simulink model "stepperMotorADRCSecondOrder"  (R2025a)
settings: Solver=FixedStepDiscrete  StartTime=0.0  StopTime=.4  FixedStep=1/50e6  RelTol=1e-3
undefined symbols (not defined in the file): ADC_Emulated_conversion_factor, alpha_iqd, alpha_ts, b_ts, beta_iqd, beta_ts, biq, Bm, DiscIntNeverNeededParam, gam_iqd, gam_ts, inverseADC_Emulated_Conversion_factor, inverseVoltagetoADCValue, J, k1_iqd, k1_ts, L, PsiM, PWMVoltage, r, RadiansPerCount, RT, Shunt_Amp_Offset, simParams, stepTime, theta_ref, TL, VoltagetoADCValue, vs
libraries: mcbeeMathTransformLib x2
settings Model: Creator=mike  LastModifiedBy=Caleb
settings OptimizationCC: BlockReduction=off  ConditionallyExecuteInputs=off  DefaultParameterBehavior=Inlined
settings HardwareCC: ProdBitPerPointer=32.0  ProdBitPerSizeT=32.0  ProdBitPerPtrDiffT=32.0  ProdLargestAtomicFloat=None  ProdIntDivRoundTo=Undefined  ProdEndianess=Unspecified  ProdWordSize=32.0  ProdHWDeviceType=ASIC/FPGA->ASIC/FPGA  TargetBitPerPointer=64.0  TargetBitPerSizeT=64.0  TargetBitPerPtrDiffT=64.0  TargetLongLongMode=on  TargetIntDivRoundTo=Zero  TargetEndianess=LittleEndian  TargetWordSize=64.0  TargetHWDeviceType=Custom Processor->MATLAB Host Computer  ProdEqTarget=off
settings RTWCC: GPUComputeCapability=3.5

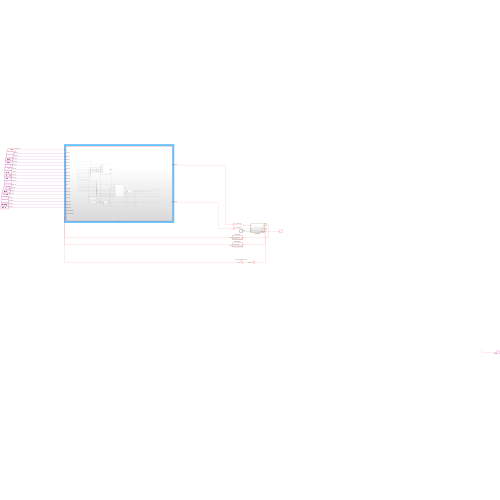
[thumbnail: Simulink's stored preview of the top-level diagram]
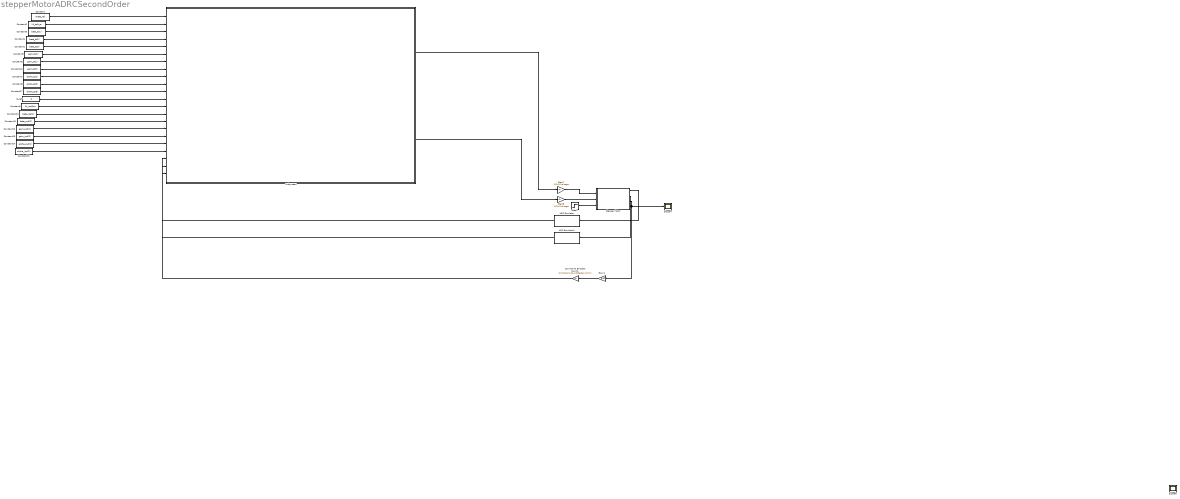
== system stepperMotorADRCSecondOrder ==
  ADC Emulator : Subsystem
  ADC Emulator1 : Subsystem
  Constant : Constant  Value=theta_ref  OutDataTypeStr=fixdt(1,16,8)  SampleTime=-1
  Constant1 : Constant  Value=beta_ts(3)  OutDataTypeStr=fixdt(1,16,8)
  Constant10 : Constant  Value=beta_iqd(1)  OutDataTypeStr=fixdt(1,16,8)
  Constant11 : Constant  Value=beta_iqd(2)  OutDataTypeStr=fixdt(1,16,8)
  Constant12 : Constant  Value=gam_iqd(1)  OutDataTypeStr=fixdt(1,16,8)
  Constant13 : Constant  Value=gam_iqd(2)  OutDataTypeStr=fixdt(1,16,8)
  Constant14 : Constant  Value=alpha_iqd(1)  OutDataTypeStr=fixdt(1,16,8)
  Constant15 : Constant  Value=alpha_iqd(2)  OutDataTypeStr=fixdt(1,16,8)
  Constant16 : Constant  Value=gam_ts(3)  OutDataTypeStr=fixdt(1,16,8)
  Constant17 : Constant  Value=alpha_ts(3)  OutDataTypeStr=fixdt(1,16,8)
  Constant2 : Constant  Value=k1_ts/b_ts  OutDataTypeStr=fixdt(1,16,8)
  Constant3 : Constant  Value=beta_ts(1)  OutDataTypeStr=fixdt(1,16,8)
  Constant4 : Constant  Value=beta_ts(2)  OutDataTypeStr=fixdt(1,16,8)
  Constant5 : Constant  Value=gam_ts(1)  OutDataTypeStr=fixdt(1,16,8)
  Constant6 : Constant  Value=gam_ts(2)  OutDataTypeStr=fixdt(1,16,8)
  Constant7 : Constant  Value=alpha_ts(1)  OutDataTypeStr=fixdt(1,16,8)
  Constant8 : Constant  Value=alpha_ts(2)  OutDataTypeStr=fixdt(1,16,8)
  Constant9 : Constant  Value=k1_iqd/biq  OutDataTypeStr=fixdt(1,16,8)
  Convert To Encoder Counts : Gain  Gain=simParams.CountsPerRev/(2*pi)  OutDataTypeStr=int32
  Gain1 : Gain  Gain=1/RT
  Gain2 : Gain  Gain=1/PWMVoltage  ParamDataTypeStr=fixdt(1,16,8)  OutDataTypeStr=fixdt(1,20,18)
  Gain3 : Gain  Gain=1/PWMVoltage  ParamDataTypeStr=fixdt(1,16,8)  OutDataTypeStr=fixdt(1,20,18)
  Scope4 : Scope
      settings: DataLoggingVariableName=ScopeData4
  Scope6 : Scope
      settings: DataLoggingVariableName=ScopeData6
  Step1 : Step  Time=stepTime  After=TL  SampleTime=0
  Stepper Motor : Subsystem
  Subsystem : Subsystem
  id_ref : Constant  Value=0  OutDataTypeStr=fixdt(1,16,8)
  wires:
  Gain1/1 -> Convert To Encoder Counts/1
  Gain2/1 -> Stepper Motor/1(va)
  Gain3/1 -> Stepper Motor/2(vb)
  Stepper Motor/3(theta_r) -> Scope4/1, Gain1/1
  Stepper Motor/2(ib) -> ADC Emulator1/1(ib)
  Step1/1 -> Stepper Motor/3(TL)
  Stepper Motor/1(ia) -> ADC Emulator/1(ia)
  ? -> Scope6/1
  Constant/1 -> Subsystem/1(r1)
  Constant2/1 -> Subsystem/2(K1_ts/b_ts)
  Constant3/1 -> Subsystem/3(beta_ts(1))
  Constant4/1 -> Subsystem/4(beta_ts(2))
  Constant1/1 -> Subsystem/5(beta_ts(3))
  Constant5/1 -> Subsystem/6(gam_ts(1))
  Constant6/1 -> Subsystem/7(gam_ts(2))
  Constant16/1 -> Subsystem/8(gam_ts(3))
  Constant7/1 -> Subsystem/9(alpha_ts(1))
  Constant8/1 -> Subsystem/10(alpha_ts(2))
  Constant17/1 -> Subsystem/11(alpha_ts(3))
  id_ref/1 -> Subsystem/12(id_ref)
  Constant9/1 -> Subsystem/13(k1_iqd/biq)
  Constant10/1 -> Subsystem/14(beta_iqd(1))
  Constant11/1 -> Subsystem/15(beta_iqd(2))
  Constant12/1 -> Subsystem/16(gam_iqd(1))
  Constant13/1 -> Subsystem/17(gam_iqd(2))
  Constant14/1 -> Subsystem/18(alpha_iqd(1))
  Constant15/1 -> Subsystem/19(alpha_iqd(2))
  ADC Emulator/1(ADC Current Value) -> Subsystem/20(ADC Current Value)
  ADC Emulator1/1(ADC Current Value) -> Subsystem/21(ADC Current Value1)
  Convert To Encoder Counts/1 -> Subsystem/22(In22)
  Subsystem/1(Out1) -> Gain2/1
  Subsystem/2(Out2) -> Gain3/1

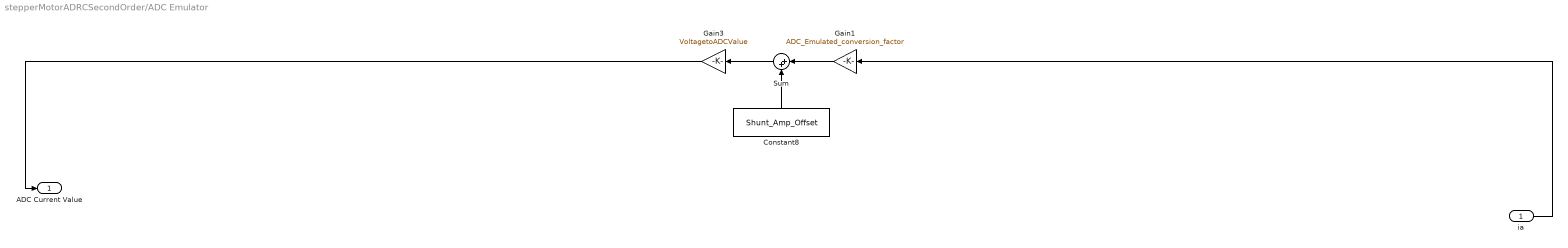
== system stepperMotorADRCSecondOrder/ADC Emulator ==
  ia : Inport
  Constant8 : Constant  Value=Shunt_Amp_Offset  OutDataTypeStr=fixdt(1,16,8)
  Gain1 : Gain  Gain=ADC_Emulated_conversion_factor  ParamDataTypeStr=fixdt(1,16,8)
  Gain3 : Gain  Gain=VoltagetoADCValue  ParamDataTypeStr=int16  OutMin=[0]  OutMax=[4095]  OutDataTypeStr=fixdt(0,16,0)
  Sum : Sum  Inputs=|++  OutDataTypeStr=Inherit: Inherit via back propagation
  ADC Current Value : Outport
  wires:
  Sum/1 -> Gain3/1
  Gain1/1 -> Sum/1
  Gain3/1 -> ADC Current Value/1
  Constant8/1 -> Sum/2
  ia/1 -> Gain1/1

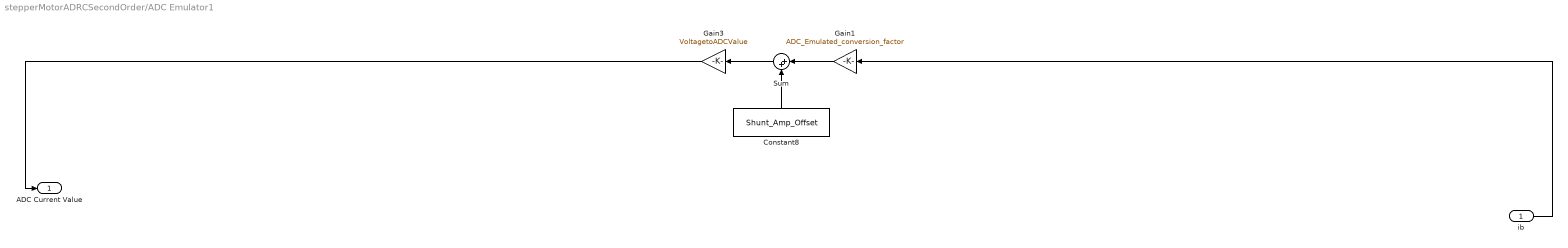
== system stepperMotorADRCSecondOrder/ADC Emulator1 ==
  ib : Inport
  Constant8 : Constant  Value=Shunt_Amp_Offset  OutDataTypeStr=fixdt(1,16,8)
  Gain1 : Gain  Gain=ADC_Emulated_conversion_factor  ParamDataTypeStr=fixdt(1,16,8)
  Gain3 : Gain  Gain=VoltagetoADCValue  ParamDataTypeStr=int16  OutMin=[0]  OutMax=[4095]  OutDataTypeStr=fixdt(0,16,0)
  Sum : Sum  Inputs=|++  OutDataTypeStr=Inherit: Inherit via back propagation
  ADC Current Value : Outport
  wires:
  Sum/1 -> Gain3/1
  Gain1/1 -> Sum/1
  Gain3/1 -> ADC Current Value/1
  Constant8/1 -> Sum/2
  ib/1 -> Gain1/1

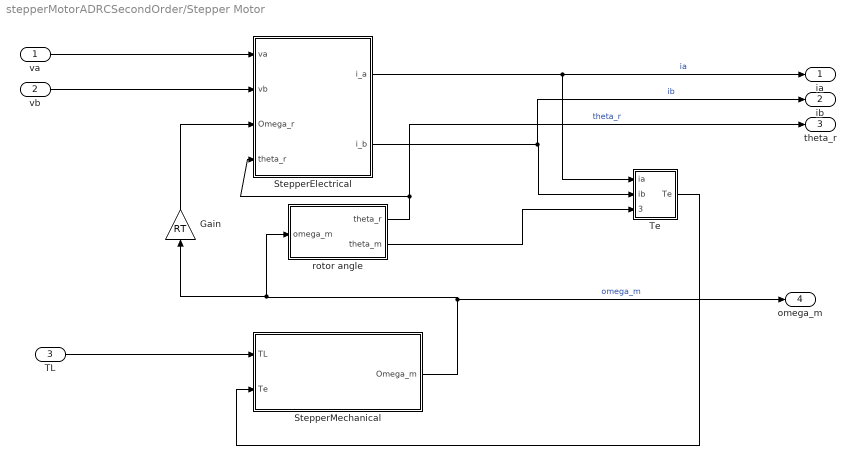
== system stepperMotorADRCSecondOrder/Stepper Motor ==
  va : Inport
  vb : Inport  Port=2
  TL : Inport  Port=3
  Gain : Gain  Gain=RT
  StepperElectrical : Subsystem
  StepperMechanical : Subsystem
  Te : Subsystem
  rotor angle : Subsystem
  ia : Outport
  ib : Outport  Port=2
  theta_r : Outport  Port=3
  omega_m : Outport  Port=4
  wires:
  va/1 -> StepperElectrical/1(va)
  vb/1 -> StepperElectrical/2(vb)
  TL/1 -> StepperMechanical/1(TL)
  Te/1(Te) -> StepperMechanical/2(Te)
  StepperMechanical/1(Omega_m) -> Gain/1, rotor angle/1(omega_m), omega_m/1  "omega_m"
  Gain/1 -> StepperElectrical/3(Omega_r)
  rotor angle/2(theta_m) -> Te/3(theta_m)
  StepperElectrical/1(i_a) -> ia/1, Te/1(ia)  "ia"
  StepperElectrical/2(i_b) -> ib/1, Te/2(ib)  "ib"
  rotor angle/1(theta_r) -> theta_r/1, StepperElectrical/4(theta_r)  "theta_r"

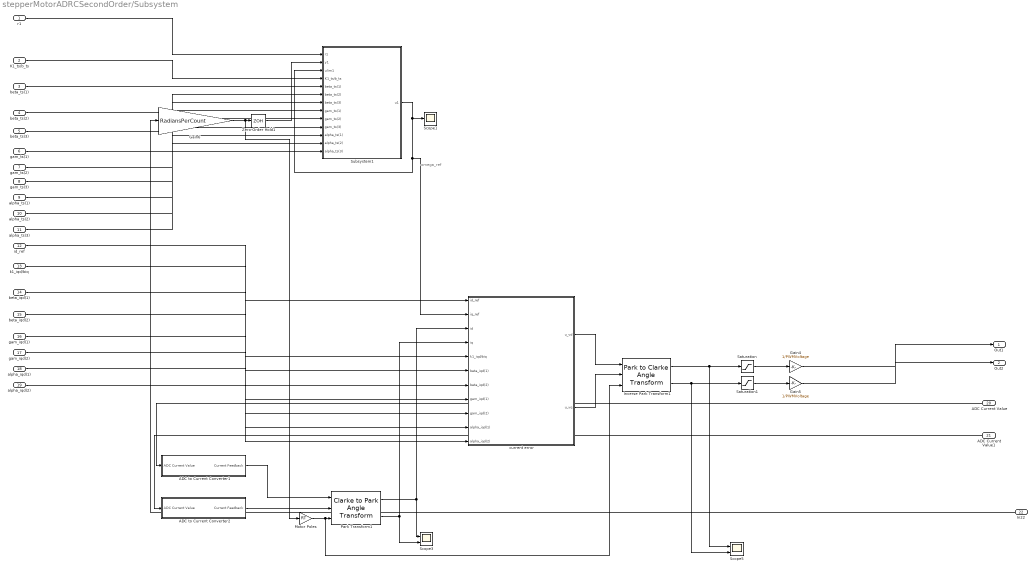
== system stepperMotorADRCSecondOrder/Subsystem ==
  note: omega_ref
  r1 : Inport
  K1_ts/b_ts : Inport  Port=2
  beta_ts(1) : Inport  Port=3
  beta_ts(2) : Inport  Port=4
  beta_ts(3) : Inport  Port=5
  gam_ts(1) : Inport  Port=6
  gam_ts(2) : Inport  Port=7
  gam_ts(3) : Inport  Port=8
  alpha_ts(1) : Inport  Port=9
  alpha_ts(2) : Inport  Port=10
  alpha_ts(3) : Inport  Port=11
  id_ref : Inport  Port=12
  k1_iqd/biq : Inport  Port=13
  beta_iqd(1) : Inport  Port=14
  beta_iqd(2) : Inport  Port=15
  gam_iqd(1) : Inport  Port=16
  gam_iqd(2) : Inport  Port=17
  alpha_iqd(1) : Inport  Port=18
  alpha_iqd(2) : Inport  Port=19
  ADC Current Value : Inport  Port=20
  ADC Current Value1 : Inport  Port=21
  In22 : Inport  Port=22
  ADC to Current Converter1 : Subsystem
  ADC to Current Converter2 : Subsystem
  Gain4 : Gain  Gain=1/PWMVoltage
  Gain5 : Gain  Gain=1/PWMVoltage
  Gain6 : Gain  Gain=RadiansPerCount  OutDataTypeStr=fixdt(1,16,8)
  Inverse Park Transform1 : mcbeeMathTransformLib/Park to Clarke Angle Transform  AxisAlignment=D-axis  UseWithEmbedded=on  PhaseInput=Two inputs  ThetaInput=Electrical position  AngleInput=Radians  N_points=1024
      settings: LibrarySourceBlock=mcbhdllib/Controls/Math Transforms/Inverse Park Transform
  Motor Poles : Gain  Gain=RT  ParamDataTypeStr=fixdt(1,16,0)  OutDataTypeStr=Inherit: Same as input
  Park Transform1 : mcbeeMathTransformLib/Clarke to Park Angle Transform  AxisAlignment=D-axis  UseWithEmbedded=on  PhaseInput=Two inputs  ThetaInput=Electrical position  AngleInput=Per-unit  N_points=1024
      settings: LibrarySourceBlock=mcbhdllib/Controls/Math Transforms/Park Transform
  Saturation : Saturate  UpperLimit=PWMVoltage  LowerLimit=-PWMVoltage
  Saturation1 : Saturate  UpperLimit=PWMVoltage  LowerLimit=-PWMVoltage
  Scope1 : Scope
      settings: ActiveDisplayYMinimum=-0.16084  ActiveDisplayYMaximum=0.20991
  Scope3 : Scope  NumInputPorts=2
      settings: ActiveDisplayYMinimum=-0.00044  ActiveDisplayYMaximum=0.00065  DataLoggingVariableName=ScopeData3
  Scope5 : Scope  NumInputPorts=2
      settings: ActiveDisplayYMinimum=-0.62668  ActiveDisplayYMaximum=0.64236  DataLoggingVariableName=ScopeData5
  Subsystem1 : Subsystem
  Zero-Order Hold1 : ZeroOrderHold  SampleTime=-1
  current error : Subsystem
  Out1 : Outport
  Out2 : Outport  Port=2
  wires:
  k1_iqd/biq/1 -> current error/5(k1_iqd/biq)
  Subsystem1/1(u1) -> Scope1/1, current error/2(iq_ref), Subsystem1/3(ulim1)
  Gain6/1 -> Motor Poles/1, Zero-Order Hold1/1
  gam_ts(1)/1 -> Subsystem1/8(gam_ts(1))
  ADC Current Value1/1 -> ADC to Current Converter2/1(ADC Current Value)
  ADC Current Value/1 -> ADC to Current Converter1/1(ADC Current Value)
  beta_ts(1)/1 -> Subsystem1/5(beta_ts(1))
  current error/2(u_vq) -> Inverse Park Transform1/2
  gam_ts(3)/1 -> Subsystem1/10(gam_ts(3))
  alpha_iqd(1)/1 -> current error/10(alpha_iqd(1))
  Inverse Park Transform1/2 -> Saturation1/1, Scope5/2
  Gain5/1 -> Out2/1
  beta_iqd(1)/1 -> current error/6(beta_iqd(1))
  Park Transform1/1 -> Scope3/1, current error/3(id)
  Inverse Park Transform1/1 -> Saturation/1, Scope5/1
  Gain4/1 -> Out1/1
  K1_ts/b_ts/1 -> Subsystem1/4(K1_ts/b_ts)
  Saturation1/1 -> Gain5/1
  Motor Poles/1 -> Inverse Park Transform1/3, Park Transform1/3
  Zero-Order Hold1/1 -> Subsystem1/2(y1)
  Park Transform1/2 -> current error/4(iq), Scope3/2
  current error/1(u_vd) -> Inverse Park Transform1/1
  alpha_ts(3)/1 -> Subsystem1/13(alpha_ts(3))
  ADC to Current Converter1/1(Current Feedback) -> Park Transform1/1
  alpha_iqd(2)/1 -> current error/11(alpha_iqd(2))
  id_ref/1 -> current error/1(id_ref)
  beta_ts(2)/1 -> Subsystem1/6(beta_ts(2))
  Saturation/1 -> Gain4/1
  ADC to Current Converter2/1(Current Feedback) -> Park Transform1/2
  gam_ts(2)/1 -> Subsystem1/9(gam_ts(2))
  beta_iqd(2)/1 -> current error/7(beta_iqd(2))
  r1/1 -> Subsystem1/1(r1)
  gam_iqd(2)/1 -> current error/9(gam_iqd(2))
  alpha_ts(2)/1 -> Subsystem1/12(alpha_ts(2))
  gam_iqd(1)/1 -> current error/8(gam_iqd(1))
  beta_ts(3)/1 -> Subsystem1/7(beta_ts(3))
  alpha_ts(1)/1 -> Subsystem1/11(alpha_ts(1))
  In22/1 -> Gain6/1

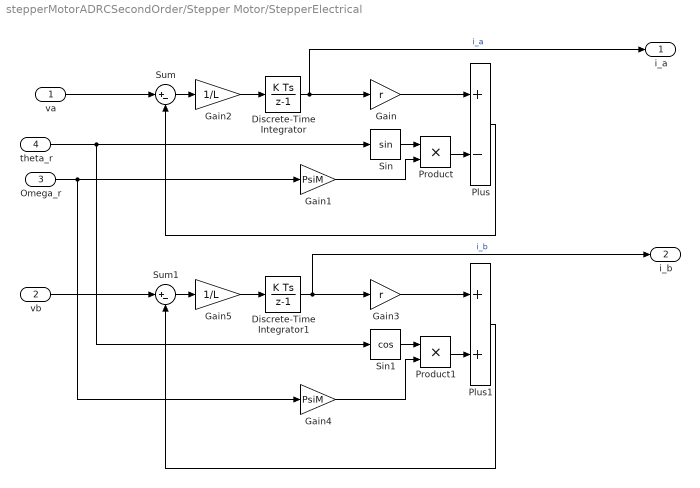
== system stepperMotorADRCSecondOrder/Stepper Motor/StepperElectrical ==
  va : Inport
  vb : Inport  Port=2
  Omega_r : Inport  Port=3
  theta_r : Inport  Port=4
  Discrete-Time Integrator : DiscreteIntegrator  SampleTime=-1  SaturateOnIntegerOverflow=on  ICPrevOutput=DiscIntNeverNeededParam  ICPrevScaledInput=DiscIntNeverNeededParam
  Discrete-Time Integrator1 : DiscreteIntegrator  SampleTime=-1  SaturateOnIntegerOverflow=on  ICPrevOutput=DiscIntNeverNeededParam  ICPrevScaledInput=DiscIntNeverNeededParam
  Gain : Gain  Gain=r
  Gain1 : Gain  Gain=PsiM
  Gain2 : Gain  Gain=1/L
  Gain3 : Gain  Gain=r
  Gain4 : Gain  Gain=PsiM
  Gain5 : Gain  Gain=1/L
  Plus : Sum  Inputs=+-
  Plus1 : Sum
  Product : Product
  Product1 : Product
  Sin : Trigonometry
  Sin1 : Trigonometry  Operator=cos
  Sum : Sum  Inputs=|+-
  Sum1 : Sum  Inputs=|+-
  i_a : Outport
  i_b : Outport  Port=2
  wires:
  va/1 -> Sum/1
  theta_r/1 -> Sin1/1, Sin/1
  Sin1/1 -> Product1/1
  Gain1/1 -> Product/2
  Plus1/1 -> Sum1/2
  vb/1 -> Sum1/1
  Gain3/1 -> Plus1/1
  Product1/1 -> Plus1/2
  Sum1/1 -> Gain5/1
  Sin/1 -> Product/1
  Discrete-Time Integrator1/1 -> i_b/1, Gain3/1  "i_b"
  Plus/1 -> Sum/2
  Gain4/1 -> Product1/2
  Gain5/1 -> Discrete-Time Integrator1/1
  Product/1 -> Plus/2
  Sum/1 -> Gain2/1
  Omega_r/1 -> Gain4/1, Gain1/1
  Gain2/1 -> Discrete-Time Integrator/1
  Gain/1 -> Plus/1
  Discrete-Time Integrator/1 -> i_a/1, Gain/1  "i_a"

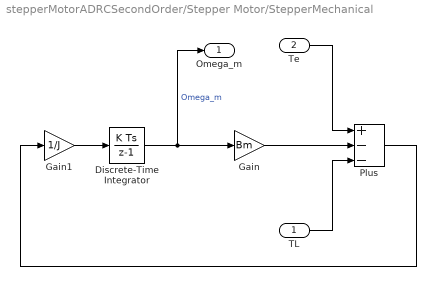
== system stepperMotorADRCSecondOrder/Stepper Motor/StepperMechanical ==
  TL : Inport
  Te : Inport  Port=2
  Discrete-Time Integrator : DiscreteIntegrator  SampleTime=-1  SaturateOnIntegerOverflow=on  ICPrevOutput=DiscIntNeverNeededParam  ICPrevScaledInput=DiscIntNeverNeededParam
  Gain : Gain  Gain=Bm
  Gain1 : Gain  Gain=1/J
  Plus : Sum  Inputs=+--
  Omega_m : Outport
  wires:
  Te/1 -> Plus/1
  Discrete-Time Integrator/1 -> Omega_m/1, Gain/1  "Omega_m"
  Gain/1 -> Plus/2
  TL/1 -> Plus/3
  Gain1/1 -> Discrete-Time Integrator/1
  Plus/1 -> Gain1/1

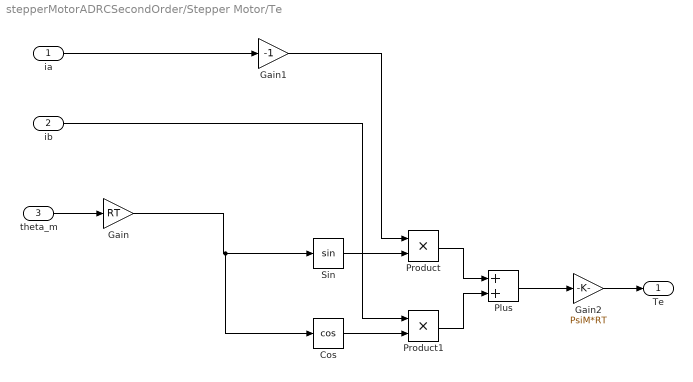
== system stepperMotorADRCSecondOrder/Stepper Motor/Te ==
  ia : Inport
  ib : Inport  Port=2
  theta_m : Inport  Port=3
  Cos : Trigonometry  Operator=cos
  Gain : Gain  Gain=RT
  Gain1 : Gain  Gain=-1
  Gain2 : Gain  Gain=PsiM*RT
  Plus : Sum
  Product : Product
  Product1 : Product
  Sin : Trigonometry
  Te : Outport
  wires:
  Gain1/1 -> Product/1
  Sin/1 -> Product/2
  Cos/1 -> Product1/2
  ib/1 -> Product1/1
  Product1/1 -> Plus/2
  ia/1 -> Gain1/1
  Product/1 -> Plus/1
  Gain2/1 -> Te/1
  Plus/1 -> Gain2/1
  theta_m/1 -> Gain/1
  Gain/1 -> Cos/1, Sin/1

== system stepperMotorADRCSecondOrder/Stepper Motor/rotor angle ==
  omega_m : Inport
  Discrete-Time Integrator : DiscreteIntegrator  SampleTime=-1  SaturateOnIntegerOverflow=on  ICPrevOutput=DiscIntNeverNeededParam  ICPrevScaledInput=DiscIntNeverNeededParam
  Gain : Gain  Gain=RT
  theta_r : Outport
  theta_m : Outport  Port=2
  wires:
  Gain/1 -> theta_r/1  "theta_r"
  omega_m/1 -> Discrete-Time Integrator/1  "omega_m"
  Discrete-Time Integrator/1 -> theta_m/1, Gain/1  "theta_m"

== system stepperMotorADRCSecondOrder/Subsystem/ADC to Current Converter1 ==
  ADC Current Value : Inport
  Constant9 : Constant  Value=Shunt_Amp_Offset  OutDataTypeStr=fixdt(1,16,8)  SampleTime=-1
  Gain : Gain  Gain=inverseADC_Emulated_Conversion_factor  OutDataTypeStr=fixdt(1,16,8)
  Gain3 : Gain  Gain=inverseVoltagetoADCValue  ParamDataTypeStr=fixdt(1,16,8)  OutDataTypeStr=fixdt(0,32,28)
  Sum3 : Sum  Inputs=|+-  OutDataTypeStr=fixdt(1,32,21)
  Current Feedback : Outport
  wires:
  ADC Current Value/1 -> Gain3/1
  Gain3/1 -> Sum3/1  "Shunt Amp Output"
  Sum3/1 -> Gain/1  "Phase A Current"
  Constant9/1 -> Sum3/2
  Gain/1 -> Current Feedback/1

== system stepperMotorADRCSecondOrder/Subsystem/ADC to Current Converter2 ==
  ADC Current Value : Inport
  Constant9 : Constant  Value=Shunt_Amp_Offset  OutDataTypeStr=fixdt(1,16,8)  SampleTime=-1
  Gain : Gain  Gain=inverseADC_Emulated_Conversion_factor  OutDataTypeStr=fixdt(1,16,8)
  Gain3 : Gain  Gain=inverseVoltagetoADCValue  ParamDataTypeStr=fixdt(1,16,8)  OutDataTypeStr=fixdt(0,32,28)
  Sum3 : Sum  Inputs=|+-  OutDataTypeStr=fixdt(1,32,21)
  Current Feedback : Outport
  wires:
  ADC Current Value/1 -> Gain3/1
  Gain3/1 -> Sum3/1  "Shunt Amp Output"
  Sum3/1 -> Gain/1  "Phase A Current"
  Constant9/1 -> Sum3/2
  Gain/1 -> Current Feedback/1

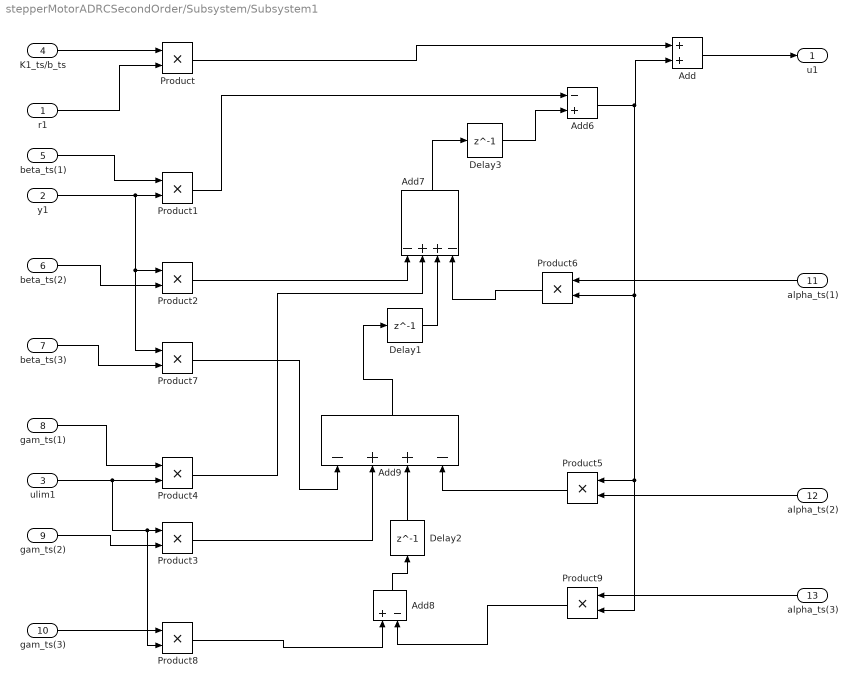
== system stepperMotorADRCSecondOrder/Subsystem/Subsystem1 ==
  r1 : Inport
  y1 : Inport  Port=2
  ulim1 : Inport  Port=3
  K1_ts/b_ts : Inport  Port=4
  beta_ts(1) : Inport  Port=5
  beta_ts(2) : Inport  Port=6
  beta_ts(3) : Inport  Port=7
  gam_ts(1) : Inport  Port=8
  gam_ts(2) : Inport  Port=9
  gam_ts(3) : Inport  Port=10
  alpha_ts(1) : Inport  Port=11
  alpha_ts(2) : Inport  Port=12
  alpha_ts(3) : Inport  Port=13
  Add : Sum  SaturateOnIntegerOverflow=on  OutDataTypeStr=Inherit: Same as first input
  Add6 : Sum  Inputs=-+  SaturateOnIntegerOverflow=on  OutDataTypeStr=Inherit: Same as first input
  Add7 : Sum  Inputs=-++-  SaturateOnIntegerOverflow=on  OutDataTypeStr=Inherit: Same as first input
  Add8 : Sum  Inputs=+-  SaturateOnIntegerOverflow=on  OutDataTypeStr=Inherit: Same as first input
  Add9 : Sum  Inputs=-++-  SaturateOnIntegerOverflow=on  OutDataTypeStr=Inherit: Same as first input
  Delay1 : Delay  DelayLength=1  InitialCondition=0
  Delay2 : Delay  DelayLength=1  InitialCondition=0
  Delay3 : Delay  DelayLength=1  InitialCondition=0
  Product{,1..9} (10 alike) : Product  SaturateOnIntegerOverflow=on  OutDataTypeStr=Inherit: Same as first input
  u1 : Outport
  wires:
  y1/1 -> Product2/1, Product7/1, Product1/2
  Product6/1 -> Add7/4
  K1_ts/b_ts/1 -> Product/1
  Product5/1 -> Add9/4
  Product3/1 -> Add9/2
  Delay3/1 -> Add6/2
  Add7/1 -> Delay3/1
  Product/1 -> Add/1
  beta_ts(2)/1 -> Product2/2
  ulim1/1 -> Product8/2, Product3/1, Product4/2
  alpha_ts(2)/1 -> Product5/2
  Add/1 -> u1/1
  r1/1 -> Product/2
  Add6/1 -> Product9/2, Product5/1, Product6/2, Add/2
  Delay1/1 -> Add7/3
  gam_ts(1)/1 -> Product4/1
  Product2/1 -> Add7/1
  Add9/1 -> Delay1/1
  Product4/1 -> Add7/2
  Product1/1 -> Add6/1
  gam_ts(2)/1 -> Product3/2
  beta_ts(1)/1 -> Product1/1
  alpha_ts(1)/1 -> Product6/1
  beta_ts(3)/1 -> Product7/2
  Product7/1 -> Add9/1
  gam_ts(3)/1 -> Product8/1
  Product8/1 -> Add8/1
  Add8/1 -> Delay2/1
  Delay2/1 -> Add9/3
  alpha_ts(3)/1 -> Product9/1
  Product9/1 -> Add8/2

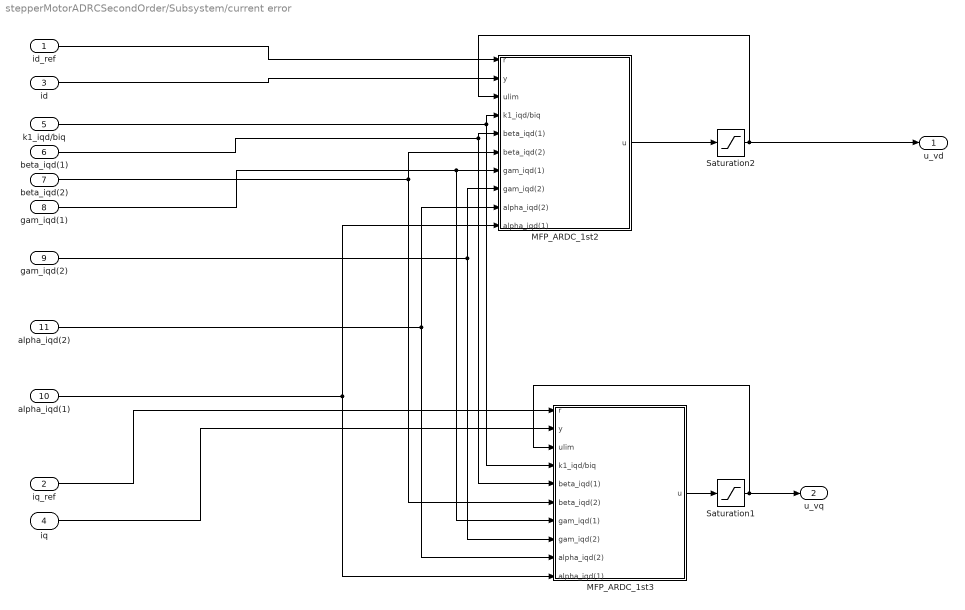
== system stepperMotorADRCSecondOrder/Subsystem/current error ==
  id_ref : Inport
  iq_ref : Inport  Port=2
  id : Inport  Port=3
  iq : Inport  Port=4
  k1_iqd/biq : Inport  Port=5
  beta_iqd(1) : Inport  Port=6
  beta_iqd(2) : Inport  Port=7
  gam_iqd(1) : Inport  Port=8
  gam_iqd(2) : Inport  Port=9
  alpha_iqd(1) : Inport  Port=10
  alpha_iqd(2) : Inport  Port=11
  MFP_ARDC_1st2 : Subsystem
  MFP_ARDC_1st3 : Subsystem
  Saturation1 : Saturate  UpperLimit=vs  LowerLimit=-vs
  Saturation2 : Saturate  UpperLimit=vs  LowerLimit=-vs
  u_vd : Outport
  u_vq : Outport  Port=2
  wires:
  iq_ref/1 -> MFP_ARDC_1st3/1(r)
  iq/1 -> MFP_ARDC_1st3/2(y)
  Saturation1/1 -> MFP_ARDC_1st3/3(ulim), u_vq/1
  MFP_ARDC_1st3/1(u) -> Saturation1/1
  id/1 -> MFP_ARDC_1st2/2(y)
  id_ref/1 -> MFP_ARDC_1st2/1(r)
  MFP_ARDC_1st2/1(u) -> Saturation2/1
  Saturation2/1 -> MFP_ARDC_1st2/3(ulim), u_vd/1
  k1_iqd/biq/1 -> MFP_ARDC_1st2/4(k1_iqd/biq), MFP_ARDC_1st3/4(k1_iqd/biq)
  beta_iqd(1)/1 -> MFP_ARDC_1st2/5(beta_iqd(1)), MFP_ARDC_1st3/5(beta_iqd(1))
  beta_iqd(2)/1 -> MFP_ARDC_1st3/6(beta_iqd(2)), MFP_ARDC_1st2/6(beta_iqd(2))
  gam_iqd(1)/1 -> MFP_ARDC_1st2/7(gam_iqd(1)), MFP_ARDC_1st3/7(gam_iqd(1))
  gam_iqd(2)/1 -> MFP_ARDC_1st2/8(gam_iqd(2)), MFP_ARDC_1st3/8(gam_iqd(2))
  alpha_iqd(2)/1 -> MFP_ARDC_1st2/9(alpha_iqd(2)), MFP_ARDC_1st3/9(alpha_iqd(2))
  alpha_iqd(1)/1 -> MFP_ARDC_1st2/10(alpha_iqd(1)), MFP_ARDC_1st3/10(alpha_iqd(1))

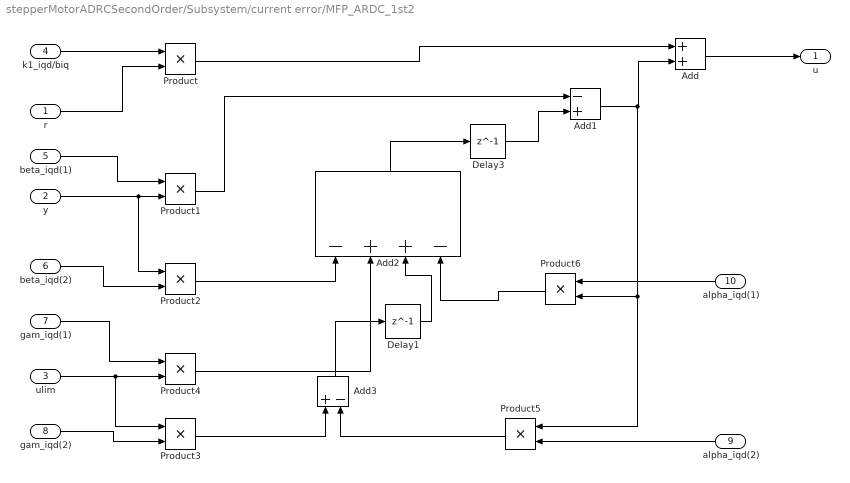
== system stepperMotorADRCSecondOrder/Subsystem/current error/MFP_ARDC_1st2 ==
  r : Inport
  y : Inport  Port=2
  ulim : Inport  Port=3
  k1_iqd/biq : Inport  Port=4
  beta_iqd(1) : Inport  Port=5
  beta_iqd(2) : Inport  Port=6
  gam_iqd(1) : Inport  Port=7
  gam_iqd(2) : Inport  Port=8
  alpha_iqd(2) : Inport  Port=9
  alpha_iqd(1) : Inport  Port=10
  Add : Sum  SaturateOnIntegerOverflow=on  OutDataTypeStr=Inherit: Same as first input
  Add1 : Sum  Inputs=-+  SaturateOnIntegerOverflow=on  OutDataTypeStr=Inherit: Same as first input
  Add2 : Sum  Inputs=-++-  SaturateOnIntegerOverflow=on  OutDataTypeStr=Inherit: Same as first input
  Add3 : Sum  Inputs=+-  SaturateOnIntegerOverflow=on  OutDataTypeStr=Inherit: Same as first input
  Delay1 : Delay  DelayLength=1  InitialCondition=0
  Delay3 : Delay  DelayLength=1  InitialCondition=0
  Product{,1..6} (7 alike) : Product  SaturateOnIntegerOverflow=on  OutDataTypeStr=Inherit: Same as first input
  u : Outport
  wires:
  Add/1 -> u/1
  Add3/1 -> Delay1/1
  Product4/1 -> Add2/2
  Product6/1 -> Add2/4
  Add1/1 -> Product5/1, Product6/2, Add/2
  Add2/1 -> Delay3/1
  r/1 -> Product/2
  Delay1/1 -> Add2/3
  Product3/1 -> Add3/1
  ulim/1 -> Product3/1, Product4/2
  Product2/1 -> Add2/1
  Product5/1 -> Add3/2
  Delay3/1 -> Add1/2
  Product1/1 -> Add1/1
  y/1 -> Product2/1, Product1/2
  k1_iqd/biq/1 -> Product/1
  Product/1 -> Add/1
  beta_iqd(1)/1 -> Product1/1
  beta_iqd(2)/1 -> Product2/2
  gam_iqd(1)/1 -> Product4/1
  gam_iqd(2)/1 -> Product3/2
  alpha_iqd(2)/1 -> Product5/2
  alpha_iqd(1)/1 -> Product6/1

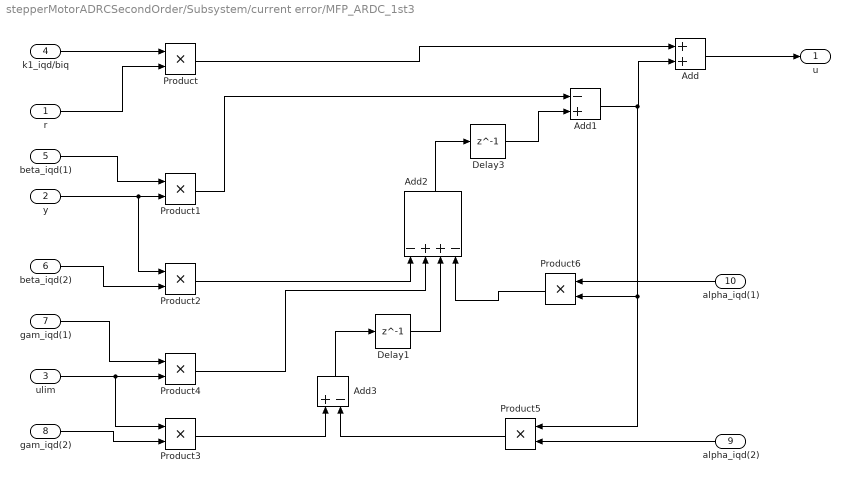
== system stepperMotorADRCSecondOrder/Subsystem/current error/MFP_ARDC_1st3 ==
  r : Inport
  y : Inport  Port=2
  ulim : Inport  Port=3
  k1_iqd/biq : Inport  Port=4
  beta_iqd(1) : Inport  Port=5
  beta_iqd(2) : Inport  Port=6
  gam_iqd(1) : Inport  Port=7
  gam_iqd(2) : Inport  Port=8
  alpha_iqd(2) : Inport  Port=9
  alpha_iqd(1) : Inport  Port=10
  Add : Sum  SaturateOnIntegerOverflow=on  OutDataTypeStr=Inherit: Same as first input
  Add1 : Sum  Inputs=-+  SaturateOnIntegerOverflow=on  OutDataTypeStr=Inherit: Same as first input
  Add2 : Sum  Inputs=-++-  SaturateOnIntegerOverflow=on  OutDataTypeStr=Inherit: Same as first input
  Add3 : Sum  Inputs=+-  SaturateOnIntegerOverflow=on  OutDataTypeStr=Inherit: Same as first input
  Delay1 : Delay  DelayLength=1  InitialCondition=0
  Delay3 : Delay  DelayLength=1  InitialCondition=0
  Product{,1..6} (7 alike) : Product  SaturateOnIntegerOverflow=on  OutDataTypeStr=Inherit: Same as first input
  u : Outport
  wires:
  Add/1 -> u/1
  Add3/1 -> Delay1/1
  Product4/1 -> Add2/2
  Product6/1 -> Add2/4
  Add1/1 -> Product5/1, Product6/2, Add/2
  Add2/1 -> Delay3/1
  r/1 -> Product/2
  Delay1/1 -> Add2/3
  Product3/1 -> Add3/1
  ulim/1 -> Product3/1, Product4/2
  Product2/1 -> Add2/1
  Product5/1 -> Add3/2
  Delay3/1 -> Add1/2
  Product1/1 -> Add1/1
  y/1 -> Product2/1, Product1/2
  k1_iqd/biq/1 -> Product/1
  Product/1 -> Add/1
  beta_iqd(1)/1 -> Product1/1
  beta_iqd(2)/1 -> Product2/2
  gam_iqd(1)/1 -> Product4/1
  gam_iqd(2)/1 -> Product3/2
  alpha_iqd(2)/1 -> Product5/2
  alpha_iqd(1)/1 -> Product6/1
